simulink model "c172_example"  (R2023b)
settings: Solver=VariableStepAuto  StartTime=0.0  StopTime=200  RelTol=1e-3
settings Model: Creator=test  LastModifiedBy=Andrea
settings SolverCC: AlgebraicLoopSolver=TrustRegion
settings DebuggingCC: UnconnectedInputMsg=warning  UnconnectedOutputMsg=warning  UnconnectedLineMsg=warning
settings ModelReferenceCC: EnableRefExpFcnMdlSchedulingChecks=on
settings RTWCC: DLArmComputeVersion=19.05

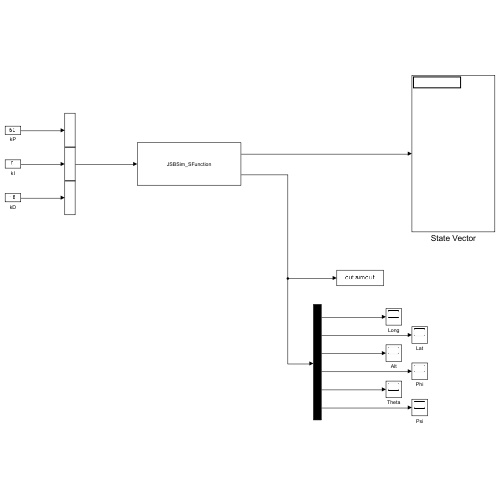
[thumbnail: Simulink's stored preview of the top-level diagram]
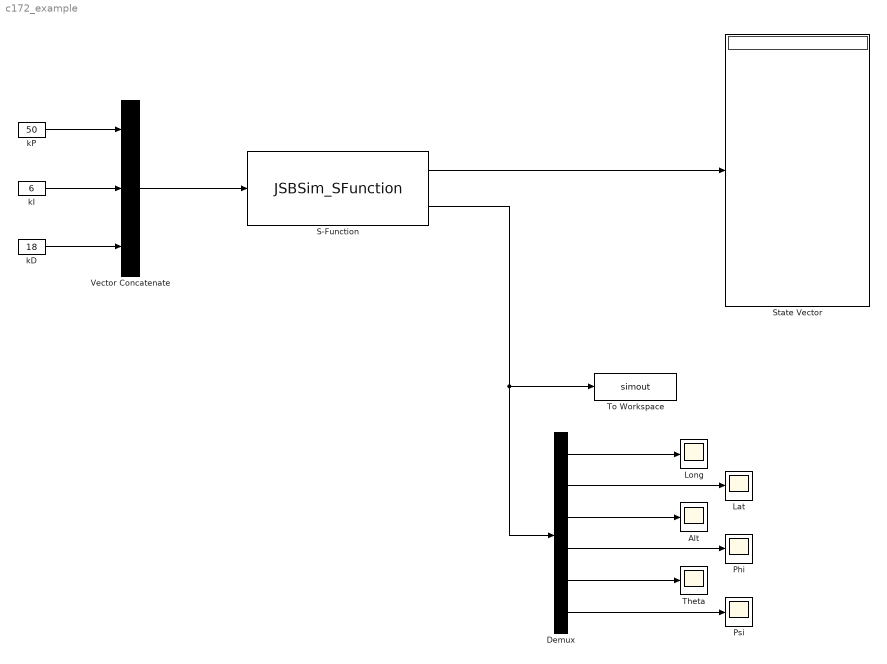
== system c172_example ==
  Alt : Scope
  Demux : Demux  Outputs=6
  Lat : Scope
  Long : Scope
  Phi : Scope
  Psi : Scope
  S-Function : S-Function  FunctionName=JSBSim_SFunction  Parameters='c172x', 0.0083333, 1, 'scripts/script_c172', 'reset01', 'io/c172_io'  SFunctionDeploymentMode=off  EnableBusSupport=off
  State Vector : Display
  Theta : Scope
  To Workspace : ToWorkspace  VariableName=simout  SaveFormat=Timeseries  SampleTime=-1
  Vector Concatenate : Concatenate  NumInputs=3
  kD : Constant  Value=18
  kI : Constant  Value=6
  kP : Constant  Value=50
  wires:
  Vector Concatenate/1 -> S-Function/1
  kD/1 -> Vector Concatenate/3
  kI/1 -> Vector Concatenate/2
  kP/1 -> Vector Concatenate/1
  S-Function/1 -> State Vector/1
  S-Function/2 -> Demux/1, To Workspace/1
  Demux/1 -> Long/1
  Demux/2 -> Lat/1
  Demux/3 -> Alt/1
  Demux/5 -> Theta/1
  Demux/4 -> Phi/1
  Demux/6 -> Psi/1
